simulink model "MagnetoShield_LQ_Simulation"  (R2019a)
settings: Solver=VariableStepAuto  StartTime=0.0  StopTime=15  RelTol=1e-3
undefined symbols (not defined in the file): A, B, C, Ck, DiscIntNeverNeededParam, Discrete, Dk, i0, K, R, sigbuilder_block, Time, Ts, u0, y0
libraries: simulink x2, ctrlSharedLib x1
settings Model: Creator=jakub  LastModifiedBy=jakub

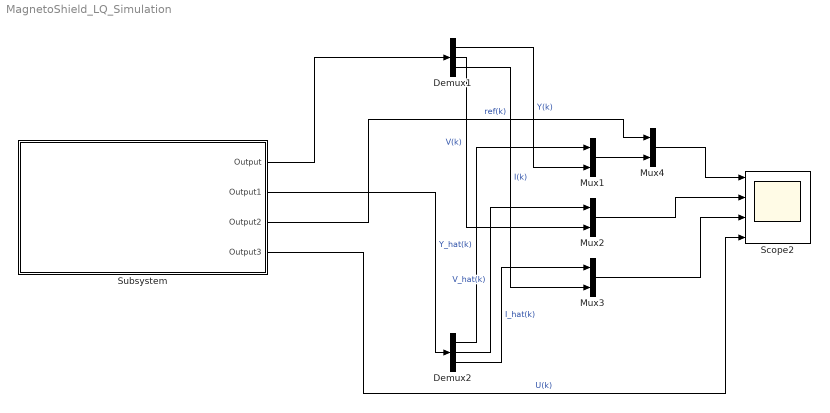
== system MagnetoShield_LQ_Simulation ==
  Demux1 : Demux  Outputs=3
  Demux2 : Demux  Outputs=3
  Mux{1..4} (4 alike) : Mux  Inputs=2
  Scope2 : Scope  NumInputPorts=4
  Subsystem : Subsystem
  wires:
  Subsystem/4(Output3) -> Scope2/4  "U(k)"
  Demux1/3 -> Mux3/2  "I(k)"
  Subsystem/2(Output1) -> Demux2/1
  Demux2/3 -> Mux3/1  "I_hat(k)"
  Subsystem/3(Output2) -> Mux4/1  "ref(k)"
  Mux1/1 -> Mux4/2
  Subsystem/1(Output) -> Demux1/1
  Demux1/2 -> Mux2/2  "V(k)"
  Mux2/1 -> Scope2/2
  Demux1/1 -> Mux1/2  "Y(k)"
  Mux3/1 -> Scope2/3
  Demux2/2 -> Mux2/1  "V_hat(k)"
  Demux2/1 -> Mux1/1  "Y_hat(k)"
  Mux4/1 -> Scope2/1

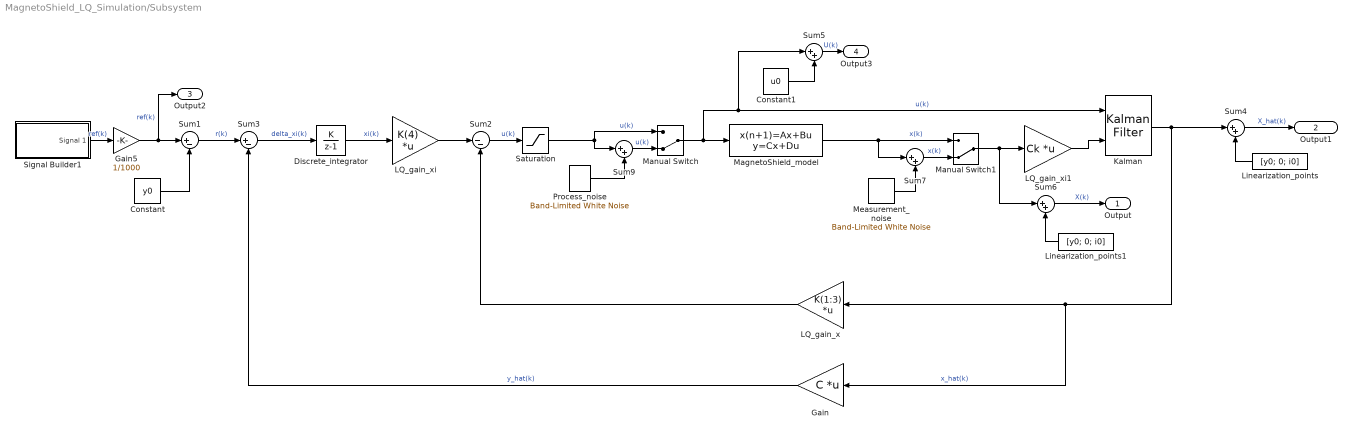
== system MagnetoShield_LQ_Simulation/Subsystem ==
  Constant : Constant  Value=y0
  Constant1 : Constant  Value=u0
  Discrete_integrator : DiscreteIntegrator  IntegratorMethod=Accumulation: Forward Euler  SampleTime=Ts  LimitOutput=on  ICPrevOutput=DiscIntNeverNeededParam  ICPrevScaledInput=DiscIntNeverNeededParam
  Gain : Gain  Gain=C  Multiplication=Matrix(K*u)
  Gain5 : Gain  Gain=1/1000
  Kalman : ctrlSharedLib/Kalman Filter  TimeDomain=Discrete-Time  UseCurrentEstimator=on  ModelSource=Individual A, B, C, D matrices  ModelSourceVariable=ss(0.95,1,1,0,1)  A=A  B=B  C=Ck  D=Dk  NumberOfStates=1  NumberOfInputs=1  NumberOfOutputs=1  InitialEstimateSource=Dialog  X0=[0.017-y0;0;0-i0]  P0=10  UseK=off  UseGH=off  NumberOfProcessNoiseInputs=1  G=1  TimeInvariantG=on  H=0  TimeInvariantH=on  Q=Q  TimeInvariantQ=on  R=R  TimeInvariantR=on  N=0  TimeInvariantN=on  AddInputPort=on  AddEnablePort=off  OutputEstimatedY=off  OutputP=off  Ts=-1
  LQ_gain_x : Gain  Gain=K(1:3)  Multiplication=Matrix(K*u)
  LQ_gain_xi : Gain  Gain=K(4)  Multiplication=Matrix(K*u)
  LQ_gain_xi1 : Gain  Gain=Ck  Multiplication=Matrix(K*u)
  Linearization_points : Constant  Value=[y0; 0; i0]
  Linearization_points1 : Constant  Value=[y0; 0; i0]
  MagnetoShield_model : DiscreteStateSpace  A=A  B=B  C=[1 0 0;0 1 0;0 0 1]  D=[0;0;0]  InitialCondition=[0.017-y0;0;0-i0]  SampleTime=Ts
  Manual Switch : ManualSwitch  CurrentSetting=0
  Manual Switch1 : ManualSwitch  CurrentSetting=0
  Measurement_noise : simulink/Sources/Band-Limited White Noise  Cov=[(6*10^(-7))^2]  Ts=2*Ts  seed=[23341]
  Process_noise : simulink/Sources/Band-Limited White Noise  Cov=[(2*10^(-3))^2]  Ts=2*Ts  seed=[23341]
  Saturation : Saturate  UpperLimit=10-u0  LowerLimit=0-u0
  Signal Builder1 : Subsystem  Tag=STV Subsys  LoadFcn=sigbuilder_block('load');  StartFcn=sigbuilder_block('start');  StopFcn=sigbuilder_block('stop');  ClipboardFcn=sigbuilder_block('clipboard');  mask(Sigbuilder block){tuvar=[0:10]}
      mask help: Simulink:masks:SigbuilderBlock_MD
      mask init:
      | if ~strcmp(get_param(bdroot(gcbh),'SimulationStatus'),'stopped') tuvar = sigbuilder_block('maskInit'); end
      settings: CopyFcn=sigbuilder_block('copy');  DeleteFcn=sigbuilder_block('delete');  ModelCloseFcn=sigbuilder_block('modelClose');  PreSaveFcn=sigbuilder_block('preSave');  PauseFcn=sigbuilder_block('pause');  ContinueFcn=sigbuilder_block('continue');  NameChangeFcn=sigbuilder_block('namechange');  OpenFcn=sigbuilder_block('open',[434.4 169.8 550.8 400.2 ]);  CloseFcn=sigbuilder_block('close');
      mask Display: plot(0, 0, 100, 100,[2, 2, 32, 32, 2], [68, 8, 8, 68, 68],[32, 2], [38, 38], [32, 19, 2],[53, 60, 44], [32, 17, 17, 2],[16, 16, 31, 31]);txt = getActiveGroup(gcbh);text(2, 100, txt,'verticalAlignment', 'top');
  Sum1 : Sum  Inputs=|+-
  Sum2 : Sum  Inputs=|--
  Sum3 : Sum  Inputs=|+-
  Sum{4..7,9} (5 alike) : Sum  Inputs=|++
  Output : Outport
  Output1 : Outport  Port=2
  Output2 : Outport  Port=3
  Output3 : Outport  Port=4
  wires:
  Sum4/1 -> Output1/1  "X_hat(k)"
  LQ_gain_x/1 -> Sum2/2
  Sum2/1 -> Saturation/1  "u(k)"
  Gain5/1 -> Output2/1, Sum1/1  "ref(k)"
  LQ_gain_xi/1 -> Sum2/1
  Sum1/1 -> Sum3/1  "r(k)"
  Kalman/1 -> Sum4/1, Gain/1, LQ_gain_x/1  "x_hat(k)"
  Manual Switch1/1 -> LQ_gain_xi1/1, Sum6/1
  Discrete_integrator/1 -> LQ_gain_xi/1  "xi(k)"
  Manual Switch/1 -> MagnetoShield_model/1, Sum5/1, Kalman/1  "u(k)"
  Linearization_points/1 -> Sum4/2
  Process_noise/1 -> Sum9/2
  Sum3/1 -> Discrete_integrator/1  "delta_xi(k)"
  Saturation/1 -> Sum9/1, Manual Switch/1  "u(k)"
  Constant1/1 -> Sum5/2
  Sum9/1 -> Manual Switch/2  "u(k)"
  Constant/1 -> Sum1/2
  Sum5/1 -> Output3/1  "U(k)"
  Gain/1 -> Sum3/2  "y_hat(k)"
  Signal Builder1/1(Signal 1) -> Gain5/1  "ref(k)"
  LQ_gain_xi1/1 -> Kalman/2
  Linearization_points1/1 -> Sum6/2
  Sum6/1 -> Output/1  "X(k)"
  MagnetoShield_model/1 -> Manual Switch1/1, Sum7/1  "x(k)"
  Sum7/1 -> Manual Switch1/2  "x(k)"
  Measurement_noise/1 -> Sum7/2

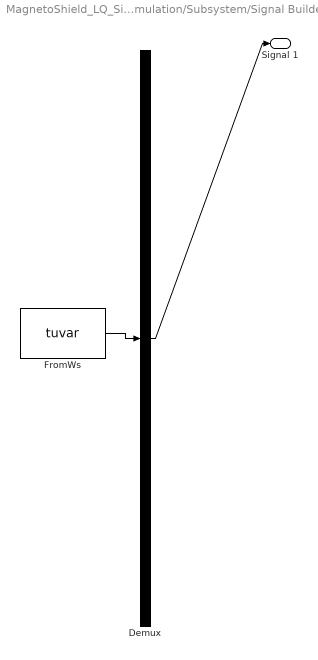
== system MagnetoShield_LQ_Simulation/Subsystem/Signal Builder1 ==
  Demux : Demux  Tag=STV Demux  Outputs=1
  FromWs : FromWorkspace  Tag=STV FromWs  VariableName=tuvar  SampleTime=0
      SigBuilderData=|
      | common.afterFinalStr = 'Extrapolate'
      | common.sampleTime = 0
      | dataSet.timeRange = [0 15]
      | dataSet.name = 'Group 1'
      | sbobj.Groups.Name = 'Group 1'
      | sbobj.Groups.Signals.Name = 'Signal 1'
      | sbobj.Groups.Signals.XData = [0 2 2 4 4 6 6 8 10 12 14 14 15]
      | sbobj.Groups.Signals.YData = [15.5 15.5 14 14 12.5 12.5 14.5 14.5 17 12 14.5 17 17]
      | sbobj.Groups.TimeRange = [0 15]
  Signal 1 : Outport  Tag=STV Outport
  wires:
  FromWs/1 -> Demux/1
  Demux/1 -> Signal 1/1
